simulink model "quad_mpc"  (R2020a)
settings: Solver=VariableStepAuto  StartTime=0.0  StopTime=10.0  RelTol=1e-3
values from neighbouring files (symbols this model uses):
  Ts = 0.1    [config_quad_mpc.m]    (also in quad_mpc_init.m)
undefined symbols (not defined in the file or in its folder): ref
libraries: mpclib x1, simulink x1
settings Model: Creator=kekatos  LastModifiedBy=kekatos
settings DebuggingCC: UnderSpecifiedDimensionMsg=warning

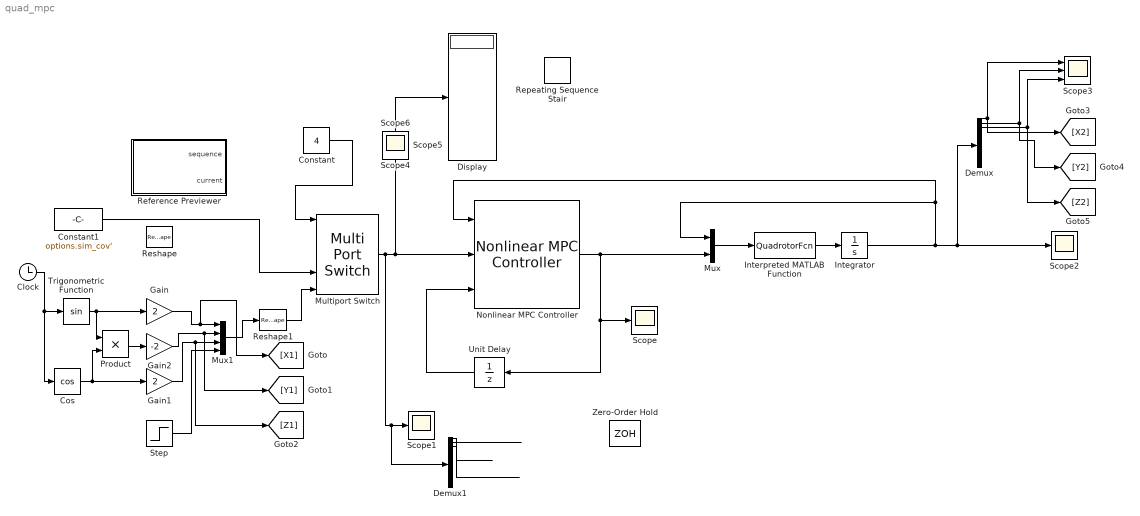
== system quad_mpc ==
  Clock : Clock
  Constant : Constant  Value=4
  Constant1 : Constant  Value=options.sim_cov'  VectorParams1D=off  SampleTime=0
  Cos : Trigonometry  Operator=cos
  Demux : Demux  Outputs=12
  Demux1 : Demux  Outputs=12
  Display : Display
  Gain : Gain  Gain=2
  Gain1 : Gain  Gain=2
  Gain2 : Gain  Gain=-2
  Integrator : Integrator
  Interpreted MATLAB Function : MATLABFcn  MATLABFcn=QuadrotorFcn  OutputDimensions=12
  Multiport Switch : MultiPortSwitch  Inputs=4
  Mux : Mux  Inputs=2
  Mux1 : Mux
  Nonlinear MPC Controller : mpclib/Nonlinear MPC Controller  SCDEnableBlockLinearizationSpecification=on  nlmpcobj=nlobj  UseObjectTs=on  UseMEX=off  md_enabled=off  mvtarget_enabled=off  param_enabled=off  cost_enabled=off  mvseq_enabled=off  stateseq_enabled=off  ovseq_enabled=off  slack_enabled=off  status_enabled=off  ov_min=off  ov_max=off  mv_min=off  mv_max=off  mvrate_min=off  mvrate_max=off  state_min=off  state_max=off  ov_weight=off  mv_weight=off  mvrate_weight=off  ecr_weight=off  nlp_initialize=off
  Product : Product
  Reference Previewer : Subsystem  mask{signal=ref, ts=Ts, steps=1}
      mask prompts: signal "Signal name"; ts "Sampling time"; steps "Number of previewing steps"
      mask init:
      | ts = evalin('base',get_param(gcbh,'ts'));
      | signal = evalin('base',get_param(gcbh,'signal'));
      | steps = evalin('base',get_param(gcbh,'steps'));
      | data = mpc_previewer_maskinit(signal,ts);
      mask Display:
      | fprintf('Future\nsample\nextractor');
      | port_label('output', 1, 'seq')
      | port_label('output', 2, '@t')
  Repeating Sequence Stair : simulink/Sources/Repeating Sequence Stair  OutValues=options.sim_cov  tsamp=options.ref_Ts  OutMin=[]  OutMax=[]  OutDataTypeStr=double  OutputDataTypeScalingMode=double  OutDataType=fixdt(0,8)  ConRadixGroup=Best Precision: Vector-wise  OutScaling=2^-12
  Reshape : Reshape  OutputDimensionality=Customize  OutputDimensions=[1,12]
  Reshape1 : Reshape  OutputDimensionality=Customize  OutputDimensions=[1,12]
  Scope{,1..2,4..6} (6 alike) : Scope
  Scope3 : Scope  NumInputPorts=3
  Step : Step  Time=0  After=[0;0;0;0;0;0;0;0;0]  SampleTime=0  VectorParams1D=off
  Trigonometric Function : Trigonometry
  Unit Delay : UnitDelay  SampleTime=-1  HasFrameUpgradeWarning=on
  Zero-Order Hold : ZeroOrderHold  SampleTime=0.01
  wires:
  Unit Delay/1 -> Nonlinear MPC Controller/3
  Constant/1 -> Multiport Switch/1
  Multiport Switch/1 -> Display/1, Nonlinear MPC Controller/2, Demux1/1, Scope1/1
  Nonlinear MPC Controller/1 -> Unit Delay/1, Scope/1, Mux/2
  Interpreted MATLAB Function/1 -> Integrator/1
  Mux/1 -> Interpreted MATLAB Function/1
  Integrator/1 -> Mux/1, Nonlinear MPC Controller/1, Demux/1, Scope2/1
  Constant1/1 -> Multiport Switch/4
  Step/1 -> Mux1/4
  Clock/1 -> Cos/1, Trigonometric Function/1
  Trigonometric Function/1 -> Product/1, Gain/1
  Gain/1 -> [X1], Mux1/1
  Cos/1 -> Product/2, Gain1/1
  Gain1/1 -> Mux1/3, [Z1]
  Product/1 -> Gain2/1
  Gain2/1 -> [Y1], Mux1/2
  Mux1/1 -> Reshape1/1
  Reshape1/1 -> Multiport Switch/5
  Demux/3 -> [Z2], Scope3/3
  Demux/1 -> [X2], Scope3/1
  Demux/2 -> [Y2], Scope3/2
  Demux1/1 -> ?
  Demux1/2 -> ?
  Demux1/3 -> ?

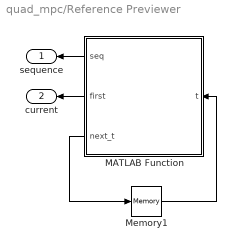
== system quad_mpc/Reference Previewer ==
  MATLAB Function : MATLAB Function  TreatAsAtomicUnit=on
  Memory1 : Memory  InheritSampleTime=on  LinearizeAsDelay=on
  sequence : Outport  VectorParamsAs1DForOutWhenUnconnected=off
  current : Outport  Port=2  VectorParamsAs1DForOutWhenUnconnected=off
  wires:
  MATLAB Function/3(next_t) -> Memory1/1
  Memory1/1 -> MATLAB Function/1(t)
  MATLAB Function/2(first) -> current/1
  MATLAB Function/1(seq) -> sequence/1

== matlab function quad_mpc/Reference Previewer/MATLAB Function ==
  settings: updateMethod=DISCRETE  sampleTime=ts
  data: data parameter; seq output; steps parameter; t input; first output; next_t output
function [seq,first,next_t] = fcn(data,steps,t)
%#codegen
[seq,first,next_t] = mpcblock_preview('ref',data,steps,t);
